simulink model "Linear_eq"  (R2024b)
settings: Solver=VariableStepAuto  StartTime=0.0  StopTime=25  RelTol=1e-3
model workspace (MAT data in the model file):
  C_yf = 30000
  C_yr = 30000
  I_zz = 2000
  l_f = 0.7
  l_r = 0.8
  m = 1000
  v_x0 = 10
settings Model: Creator=tmddn  LastModifiedBy=tmddn

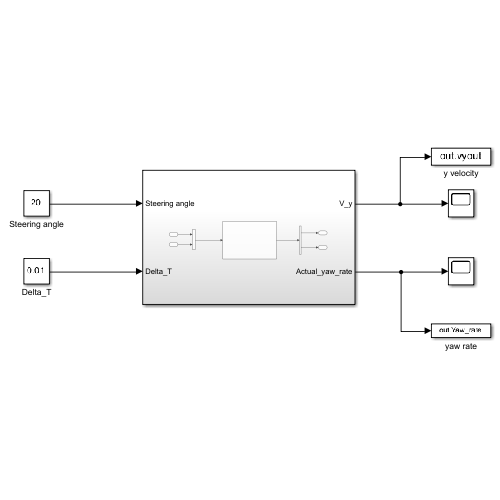
[thumbnail: Simulink's stored preview of the top-level diagram]
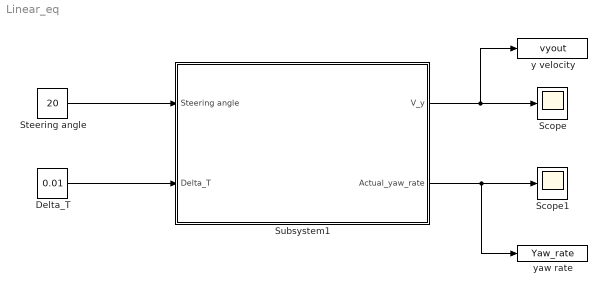
== system Linear_eq ==
  Delta_T : Constant  Value=0.01
  Scope : Scope
  Scope1 : Scope
  Steering angle : Constant  Value=20
  Subsystem1 : Subsystem
  y velocity : ToWorkspace  VariableName=vyout  SaveFormat=Timeseries  SampleTime=-1
  yaw rate : ToWorkspace  VariableName=Yaw_rate  SaveFormat=Timeseries  SampleTime=-1
  wires:
  Delta_T/1 -> Subsystem1/2(Delta_T)
  Subsystem1/2(Actual_yaw_rate) -> yaw rate/1, Scope1/1
  Steering angle/1 -> Subsystem1/1(Steering angle)
  Subsystem1/1(V_y) -> y velocity/1, Scope/1

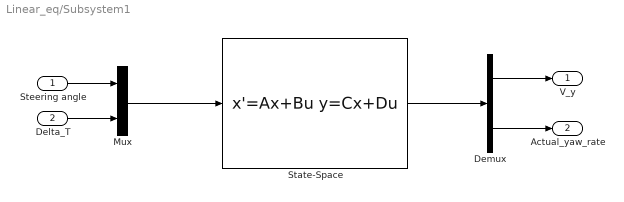
== system Linear_eq/Subsystem1 ==
  Steering angle : Inport
  Delta_T : Inport  Port=2
  Demux : Demux  Outputs=2
  Mux : Mux  Inputs=2
  State-Space : StateSpace  Priority=2  A=[-(C_yf + C_yr)/(m*v_x0), -(l_f*C_yf + l_r*C_yr)/(m*v_x0) - v_x0; -(l_f*C_yf + l_r*C_yr)/(I_zz*v_x0), -(l_f^2*C_yf + l_r^2*C_yr)/(I_zz*v_x0)]  B=[C_yf/(m*v_x0), 0; l_f*C_yf/I_zz, 1/(0.05*I_zz)]  C=[1 0; 0 1]  D=[0 0; 0 0]  InitialCondition=[0; 0]
  V_y : Outport
  Actual_yaw_rate : Outport  Port=2
  wires:
  Mux/1 -> State-Space/1
  Delta_T/1 -> Mux/2
  State-Space/1 -> Demux/1
  Steering angle/1 -> Mux/1
  Demux/1 -> V_y/1
  Demux/2 -> Actual_yaw_rate/1
